simulink model "receiver"  (R2014a)
settings: Solver=ode45  StartTime=0.0  StopTime=1  RelTol=1e-3
values from neighbouring files (symbols this model uses):
  FrameTime_CP = 4e-06    [Ofdm_Parameters.mat]
  qpsktxrxOFDM =     [Ofdm_Parameters.mat]
libraries: commdigbbndam3 x2, simulink x1, commcrc2 x1, commblkintrlv2 x1, commsdrhw_v2 x1, dspsrcs4 x1
settings Model: Creator=root  LastModifiedBy=root

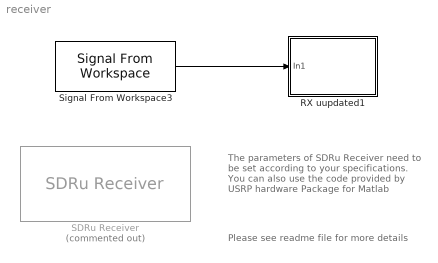
== system receiver ==
  note: Please see readme file for more details
  note: The parameters of SDRu Receiver need to be set according to your specifications. You can also use the code provided by USRP hardware Package for Matlab
  RX uupdated1 : Subsystem
      mask Display: disp('ReCeIvEr')
  SDRu Receiver : commsdrhw_v2/SDRu Receiver  Commented=on  rxtx=rx  USRP2_IP='192.168.10.2'  centerFrequency=2.45e9  centerFrequencySrc=Dialog  loOffset=0  loOffsetSrc=Dialog  gain=32  gainSrc=Dialog  decimInterp=512  decimInterpSrc=Dialog  USRP2_IP_NUM=[49 57 50 46 49 54 56 46 49 48 46 50]  frameLength=362  outputDatatype=int16  overrunUnderrunPort=off  sampleTime=1  HOST_DATA_PORT=0  HOST_CONTROL_PORT=0  USRP2_DATA_PORT=0  USRP2_CONTROL_PORT=0  bufferMode=Continuous streaming  EnableBurstMode=off  NumFramesInBurst=100
  Signal From Workspace3 : dspsrcs4/Signal From Workspace  X=corupt  Ts=2*FrameTime_CP/(qpsktxrxOFDM.OfdmSymbolSize)  nsamps=qpsktxrxOFDM.OfdmSymbolSize  OutputAfterFinalValue=Cyclic repetition  ignoreOrWarnInputAndFrameLengths=off
  wires:
  Signal From Workspace3/1 -> RX uupdated1/1(In1)

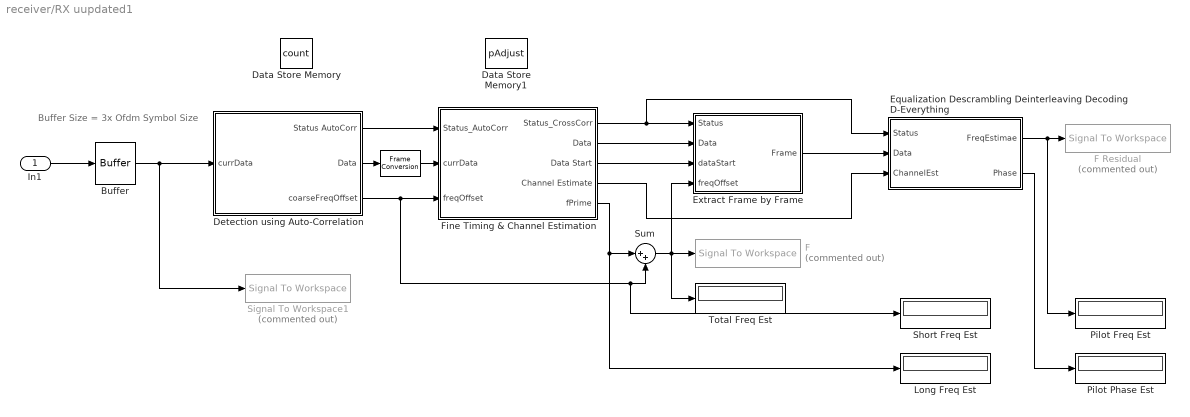
== system receiver/RX uupdated1 ==
  note: Buffer Size = 3x Ofdm Symbol Size
  In1 : Inport
  " " : FrameConversion
  Buffer : Buffer  N=qpsktxrxOFDM.OfdmSymbolSize * 3  V=qpsktxrxOFDM.OfdmSymbolSize * 2  TreatMby1Signals=One channel
  Data Store Memory : DataStoreMemory  DataStoreName=count  OutMin=0  OutMax=qpsktxrxOFDM.CounterLimit  OutDataTypeStr=double
  Data Store Memory1 : DataStoreMemory  DataStoreName=pAdjust  OutMin=0  OutMax=16  OutDataTypeStr=double
  Detection using Auto-Correlation : Subsystem
  Equalization Descrambling Deinterleaving Decoding D-Everything : Subsystem
  Extract Frame by Frame : Subsystem
  F : SignalToWorkspace  Commented=on  VariableName=freqEstTotal
      settings: CopyFcn=dspblkcopystw(gcbh);
  F Residual : SignalToWorkspace  Commented=on  VariableName=freqEstPilot
      settings: CopyFcn=dspblkcopystw(gcbh);
  Fine Timing & Channel Estimation : Subsystem
  Long Freq Est : Display
  Pilot Freq Est : Display
  Pilot Phase Est : Display
  Short Freq Est : Display
  Signal To Workspace1 : SignalToWorkspace  Commented=on  VariableName=xxx
      settings: CopyFcn=dspblkcopystw(gcbh);  Save2DSignal=3-D array (concatenate along third dimension)
  Sum : Sum  Inputs=|++
  Total Freq Est : Display
  wires:
  In1/1 -> Buffer/1
  Detection using Auto-Correlation/1(Status AutoCorr) -> Fine Timing & Channel Estimation/1(Status_AutoCorr)
  Detection using Auto-Correlation/2(Data) -> " "/1
  Buffer/1 -> Signal To Workspace1/1, Detection using Auto-Correlation/1(currData)
  " "/1 -> Fine Timing & Channel Estimation/2(currData)
  Fine Timing & Channel Estimation/2(Data) -> Extract Frame by Frame/2(Data)
  Fine Timing & Channel Estimation/3(Data Start) -> Extract Frame by Frame/3(dataStart)
  Extract Frame by Frame/1(Frame) -> Equalization Descrambling Deinterleaving Decoding D-Everything/2(Data)
  Fine Timing & Channel Estimation/4(Channel Estimate) -> Equalization Descrambling Deinterleaving Decoding D-Everything/3(ChannelEst)
  Fine Timing & Channel Estimation/1(Status_CrossCorr) -> Extract Frame by Frame/1(Status), Equalization Descrambling Deinterleaving Decoding D-Everything/1("Status ")
  Fine Timing & Channel Estimation/5(fPrime) -> Sum/1, Long Freq Est/1
  Detection using Auto-Correlation/3(coarseFreqOffset) -> Short Freq Est/1, Sum/2, Fine Timing & Channel Estimation/3(freqOffset)
  Equalization Descrambling Deinterleaving Decoding D-Everything/2(Phase) -> Pilot Phase Est/1
  Equalization Descrambling Deinterleaving Decoding D-Everything/1(FreqEstimae) -> F Residual/1, Pilot Freq Est/1
  Sum/1 -> Total Freq Est/1, F/1, Extract Frame by Frame/4(freqOffset)

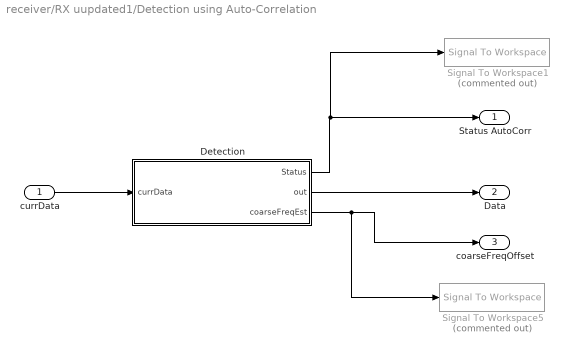
== system receiver/RX uupdated1/Detection using Auto-Correlation ==
  currData : Inport
  Detection : MATLAB Function
  Signal To Workspace1 : SignalToWorkspace  Commented=on  VariableName=StatusAutoCorr
      settings: CopyFcn=dspblkcopystw(gcbh);
  Signal To Workspace5 : SignalToWorkspace  Commented=on  VariableName=FreqEst
      settings: CopyFcn=dspblkcopystw(gcbh);
  Status AutoCorr : Outport
  Data : Outport  Port=2
  coarseFreqOffset : Outport  Port=3
  wires:
  Detection/3(coarseFreqEst) -> coarseFreqOffset/1, Signal To Workspace5/1
  Detection/1(Status) -> Signal To Workspace1/1, Status AutoCorr/1
  Detection/2(out) -> Data/1
  currData/1 -> Detection/1(currData)

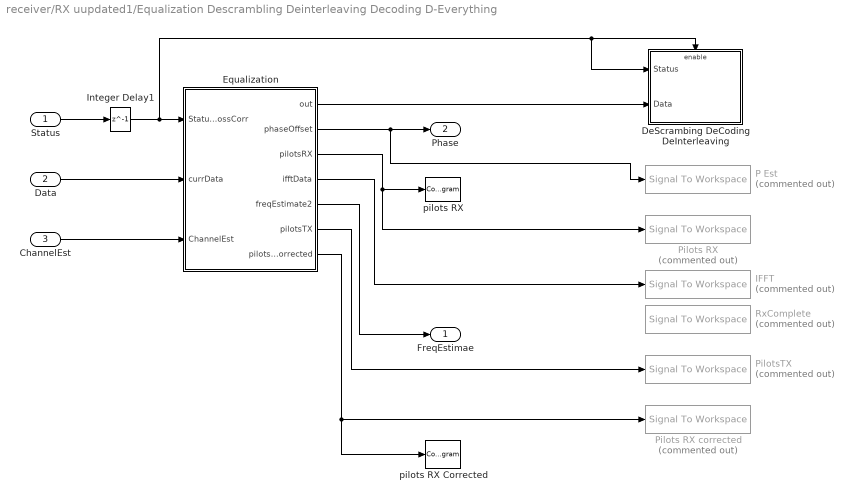
== system receiver/RX uupdated1/Equalization Descrambling Deinterleaving Decoding D-Everything ==
  "Status " : Inport
  Data : Inport  Port=2
  ChannelEst : Inport  Port=3
  DeScrambing DeCoding DeInterleaving : Subsystem
  Equalization : MATLAB Function
  IFFT : SignalToWorkspace  Commented=on  VariableName=iFFtData
      settings: CopyFcn=dspblkcopystw(gcbh);  Save2DSignal=3-D array (concatenate along third dimension)
  Integer Delay1 : Delay  DelayLength=1  InputProcessing=Inherited
  P Est : SignalToWorkspace  Commented=on  VariableName=phaseEst
      settings: CopyFcn=dspblkcopystw(gcbh);
  Pilots RX : SignalToWorkspace  Commented=on  VariableName=pilotsRX
      settings: CopyFcn=dspblkcopystw(gcbh);
  Pilots RX corrected : SignalToWorkspace  Commented=on  VariableName=pilotsRX1
      settings: CopyFcn=dspblkcopystw(gcbh);
  PilotsTX : SignalToWorkspace  Commented=on  VariableName=pilotsTX
      settings: CopyFcn=dspblkcopystw(gcbh);
  RxComplete : SignalToWorkspace  Commented=on  VariableName=RxComplete
      settings: CopyFcn=dspblkcopystw(gcbh);  Save2DSignal=3-D array (concatenate along third dimension)
  pilots RX : ConstellationDiagram  Tag=ScatterPlot
  pilots RX Corrected : ConstellationDiagram  Tag=ScatterPlot
  FreqEstimae : Outport
  Phase : Outport  Port=2
  wires:
  ChannelEst/1 -> Equalization/3(ChannelEst)
  Data/1 -> Equalization/2(currData)
  "Status "/1 -> Integer Delay1/1
  Integer Delay1/1 -> DeScrambing DeCoding DeInterleaving/1(Status), DeScrambing DeCoding DeInterleaving/Enable, Equalization/1(Status_CrossCorr)
  Equalization/2(phaseOffset) -> Phase/1, P Est/1
  Equalization/3(pilotsRX) -> Pilots RX/1, pilots RX/1
  Equalization/6(pilotsTX) -> PilotsTX/1
  Equalization/7(pilotsRX_corrected) -> Pilots RX corrected/1, pilots RX Corrected/1
  Equalization/4(ifftData) -> IFFT/1
  Equalization/1(out) -> DeScrambing DeCoding DeInterleaving/2(Data)
  ? -> RxComplete/1
  Equalization/5(freqEstimate2) -> FreqEstimae/1

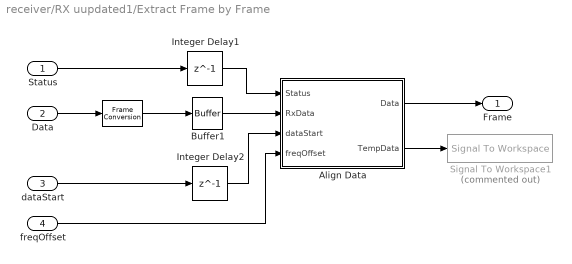
== system receiver/RX uupdated1/Extract Frame by Frame ==
  Status : Inport
  Data : Inport  Port=2
  dataStart : Inport  Port=3
  freqOffset : Inport  Port=4
  " " : FrameConversion
  Align Data : MATLAB Function  TreatAsAtomicUnit=on
  Buffer1 : Buffer  N=qpsktxrxOFDM.OfdmSymbolSize * 3  TreatMby1Signals=One channel
  Integer Delay1 : Delay  DelayLength=1  InputProcessing=Inherited
  Integer Delay2 : Delay  DelayLength=1  InputProcessing=Inherited
  Signal To Workspace1 : SignalToWorkspace  Commented=on  VariableName=TempData
      settings: CopyFcn=dspblkcopystw(gcbh);  Save2DSignal=3-D array (concatenate along third dimension)
  Frame : Outport
  wires:
  Align Data/1(Data) -> Frame/1
  Data/1 -> " "/1
  " "/1 -> Buffer1/1
  dataStart/1 -> Integer Delay2/1
  Status/1 -> Integer Delay1/1
  Integer Delay1/1 -> Align Data/1(Status)
  Buffer1/1 -> Align Data/2(RxData)
  freqOffset/1 -> Align Data/4(freqOffset)
  Align Data/2(TempData) -> Signal To Workspace1/1
  Integer Delay2/1 -> Align Data/3(dataStart)

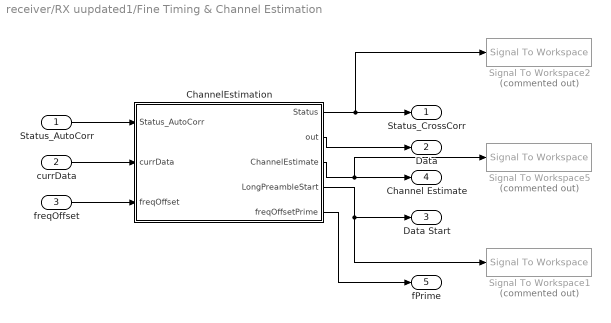
== system receiver/RX uupdated1/Fine Timing & Channel Estimation ==
  Status_AutoCorr : Inport
  currData : Inport  Port=2
  freqOffset : Inport  Port=3
  ChannelEstimation : MATLAB Function
  Signal To Workspace1 : SignalToWorkspace  Commented=on  VariableName=DataStart
      settings: CopyFcn=dspblkcopystw(gcbh);
  Signal To Workspace2 : SignalToWorkspace  Commented=on  VariableName=StatusCrossCorr
      settings: CopyFcn=dspblkcopystw(gcbh);
  Signal To Workspace5 : SignalToWorkspace  Commented=on  VariableName=ChannelESt
      settings: CopyFcn=dspblkcopystw(gcbh);
  Status_CrossCorr : Outport
  Data : Outport  Port=2
  Data Start : Outport  Port=3
  Channel Estimate : Outport  Port=4
  fPrime : Outport  Port=5
  wires:
  currData/1 -> ChannelEstimation/2(currData)
  ChannelEstimation/2(out) -> Data/1
  ChannelEstimation/1(Status) -> Status_CrossCorr/1, Signal To Workspace2/1
  Status_AutoCorr/1 -> ChannelEstimation/1(Status_AutoCorr)
  ChannelEstimation/3(ChannelEstimate) -> Signal To Workspace5/1, Channel Estimate/1
  ChannelEstimation/4(LongPreambleStart) -> Data Start/1, Signal To Workspace1/1
  freqOffset/1 -> ChannelEstimation/3(freqOffset)
  ChannelEstimation/5(freqOffsetPrime) -> fPrime/1

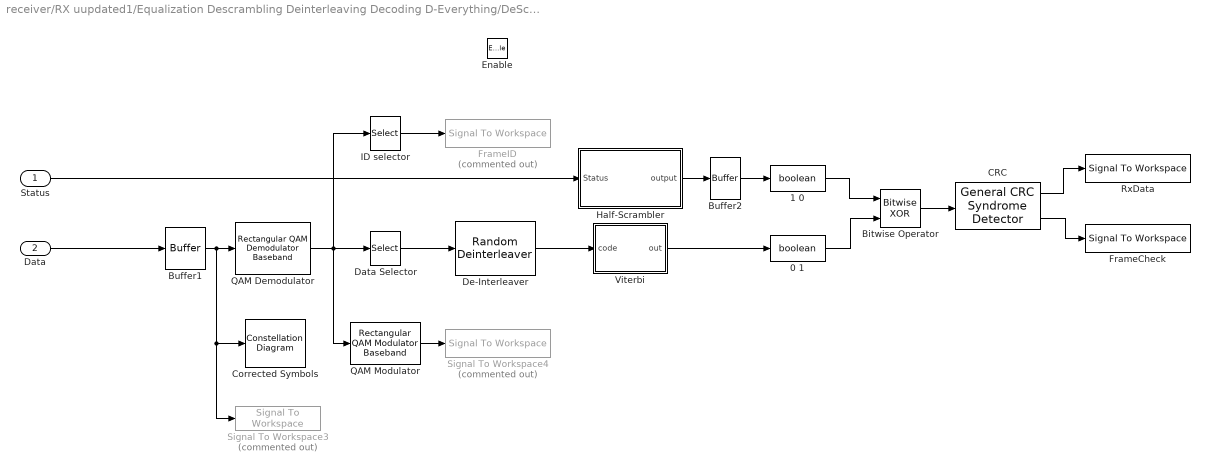
== system receiver/RX uupdated1/Equalization Descrambling Deinterleaving Decoding D-Everything/DeScrambing DeCoding DeInterleaving ==
  Status : Inport
  Data : Inport  Port=2
  Enable : EnablePort
  " QAM Modulator " : commdigbbndam3/Rectangular QAM Modulator Baseband  M=qpsktxrxOFDM.M  InType=Bit  Enc=Gray  Mapping=[0:15]  PowType=Average Power  MinDist=2  AvgPow=1  PeakPow=1  Ph=0  outDtype=double  outWordLen=16  outUDDataType=sfix(16)  outFracLenMode=Best precision  outFracLen=15
  0 1 : DataTypeConversion  OutDataTypeStr=boolean
  1 0 : DataTypeConversion  OutDataTypeStr=boolean
  Bitwise Operator : simulink/Logic and Bit Operations/Bitwise Operator  logicop=XOR  UseBitMask=off  NumInputPorts=2  BitMask=bin2dec('11011001')  BitMaskRealWorld=Stored Integer
  Buffer1 : Buffer  N=48*2  TreatMby1Signals=One channel
  Buffer2 : Buffer  N=186  TreatMby1Signals=One channel
  CRC : commcrc2/General CRC Syndrome Detector  genPoly=[1 0 0 0 0 0 0 0 1 1 1 1 1]  iniStates=0  directMethod=off  reflectInputBytes=off  reflectChecksums=off  finalXOR=0  numChecksums=1
  Corrected Symbols : ConstellationDiagram  Tag=ScatterPlot
  Data Selector : Selector  Indices=13:384
  De-Interleaver : commblkintrlv2/Random Deinterleaver  N=(qpsktxrxOFDM.DataLength + qpsktxrxOFDM.CRCLength ) * qpsktxrxOFDM.CodeRate  seed=12345
  FrameCheck : SignalToWorkspace  VariableName=FrameCheck
      settings: CopyFcn=dspblkcopystw(gcbh);
  FrameID : SignalToWorkspace  Commented=on  VariableName=FameID
      settings: CopyFcn=dspblkcopystw(gcbh);  Save2DSignal=3-D array (concatenate along third dimension)
  Half-Scrambler : MATLAB Function  TreatAsAtomicUnit=on
  ID selector : Selector  Indices=1:12
  "QAM Demodulator " : commdigbbndam3/Rectangular QAM Demodulator Baseband  M=qpsktxrxOFDM.M  PowType=Average Power  MinDist=2  AvgPow=1  PeakPow=1  Ph=0  Dec=Gray  Mapping=[0:15]  OutType=Bit  DecType=Hard decision  VarSource=Dialog  Variance=1  outDtype1=Inherit via internal rule  outDtype2=Inherit via internal rule  derotateFactorWordLen=16  denormFactorWordLen=16  prodOutWordLen=32  prodOutRoundingMode=Floor  prodOutOverflowMode=Wrap  sumWordLen=32
  RxData : SignalToWorkspace  VariableName=RxData
      settings: CopyFcn=dspblkcopystw(gcbh);  Save2DSignal=3-D array (concatenate along third dimension)
  Signal To Workspace3 : SignalToWorkspace  Commented=on  VariableName=DataSymbols
      settings: CopyFcn=dspblkcopystw(gcbh);  Save2DSignal=3-D array (concatenate along third dimension)
  Signal To Workspace4 : SignalToWorkspace  Commented=on  VariableName=DataSymbols1
      settings: CopyFcn=dspblkcopystw(gcbh);  Save2DSignal=3-D array (concatenate along third dimension)
  Viterbi : MATLAB Function  TreatAsAtomicUnit=on
  wires:
  Status/1 -> Half-Scrambler/1(Status)
  " QAM Modulator "/1 -> Signal To Workspace4/1
  "QAM Demodulator "/1 -> Data Selector/1, ID selector/1, " QAM Modulator "/1
  CRC/2 -> FrameCheck/1
  Data/1 -> Buffer1/1
  CRC/1 -> RxData/1
  Buffer1/1 -> Signal To Workspace3/1, Corrected Symbols/1, "QAM Demodulator "/1
  ID selector/1 -> FrameID/1
  Data Selector/1 -> De-Interleaver/1
  De-Interleaver/1 -> Viterbi/1(code)
  Half-Scrambler/1(output) -> Buffer2/1
  Viterbi/1(out) -> 0 1/1
  Bitwise Operator/1 -> CRC/1
  Buffer2/1 -> 1 0/1
  0 1/1 -> Bitwise Operator/2
  1 0/1 -> Bitwise Operator/1

== matlab function receiver/RX uupdated1/Fine Timing & Channel Estimation/ChannelEstimation ==
  data: Status_AutoCorr input; Status output; currData input; freqOffset input; out output; ChannelEstimate output; LongPreambleStart output; qpsktxrxOFDM parameter; count data_store_memory; freqOffsetPrime output; pAdjust data_store_memory
function [Status , out , ChannelEstimate , LongPreambleStart , freqOffsetPrime ] = channelEstimation( Status_AutoCorr , currData , freqOffset , qpsktxrxOFDM)
% THE SHORT PREAMBLES IN THE SOUBDING FRAME ARE FOLLOWED BY 10 LONG
% PREAMBLES. THE LONG PREAMBLES ARE USED FIRST TO CALCULATE REFINED START
% OF THE PACKET. CHANNEL ESTIMATE IS ALSO CALCULATED BY THE LONG PREAMBLES.
% A MORE REFINED FREQUENCY OFFSET IS ALSO CALCULATED WITH THE HELP OF LONG
% PREAMBLES.


global count pAdjust;
persistent  Status_CrossCorr ChannelEst LongPreambleStart_Est numPreambles lastPreamble endingPhase freqOffset2 freqOffsetTemp RxLongPrev;                           % No of symbols since detection

if isempty(Status_CrossCorr)
    Status_CrossCorr = 0;
    LongPreambleStart_Est = 0;
    numPreambles = 0;
    lastPreamble = 0;

    endingPhase = 0;
    freqOffset2 = 0;
    freqOffsetTemp = 0;
    RxLongPrev = complex(zeros(64,1));
end

if isempty(ChannelEst)
    ChannelEst = complex( ones(qpsktxrxOFDM.NumSubCarriers,1) );
end

if (count == qpsktxrxOFDM.CounterLimit*2)                               % time for next preambles
    count = 0;
end



% variables
longPreamble_length = 64;
Length = qpsktxrxOFDM.OfdmSymbolSize * 3; %numel(currData)


 currData2 = currData;


MaximumIndex = 0;
SecondMaximumIndex = 0;
ThirdMaximumIndex = 0;

%% PRecise Timinng via XCORR
if ( (Status_AutoCorr) && (count < 4) && (~Status_CrossCorr) ) % why equality?? 

  
    freqOffset2 = 0;
    freq = exp(1i*( 2*pi*freqOffset*(0:239).' + endingPhase ) );
    endingPhase = angle( freq(81) );
    currData = currData.*freq;
    
    ExtractedLongPreamble = qpsktxrxOFDM.Preamble(161 : 224);
    
    %% Cross Correlation    
    num_crossCorr = Length - longPreamble_length+1 ;
    CrossCorr_array = complex( zeros(1,num_crossCorr) );

    for i=1:num_crossCorr
        CrossCorr_array(i) = sum( currData(i : i + longPreamble_length - 1 ).*conj( ExtractedLongPreamble ) )...
            / sqrt( sum( ExtractedLongPreamble.*conj( ExtractedLongPreamble ) ) ...
            * sum( currData(i : i + longPreamble_length - 1 ).*conj( currData(i : i + longPreamble_length - 1 ) ) ) );
    end
    CrossCorr_array2 = abs(CrossCorr_array);
    plot(CrossCorr_array2);

    %% Checking Process
    
    [MaximumValue, MaximumIndex] = max(CrossCorr_array2);

    if (MaximumValue > .6)
    
        CrossCorr_array2 = CrossCorr_array2/MaximumValue;

        MaximumValue = 1;

        maxValue = 1;
        
        Threshold3 = 0.9;                   % detect the number of peaks
        myNumPeak=0;                        % the num of peaks in first buffer length 
        % 3 peaks and 1st maximum
        if (MaximumIndex + 64 <= 177) && (MaximumIndex + 128 <= 177) && (CrossCorr_array2(MaximumIndex + 64) >= Threshold3) && (CrossCorr_array2(MaximumIndex + 128) >= Threshold3)
            SecondMaximumIndex = MaximumIndex+64;
            SecondMaximumValue = CrossCorr_array2(SecondMaximumIndex);
            ThirdMaximumIndex = MaximumIndex+128;
            ThirdMaximumValue = CrossCorr_array2(ThirdMaximumIndex);
            myNumPeak=3;
            
            
        % 3 peaks and 2nd maximum
        elseif (MaximumIndex + 64 <= 177) && (MaximumIndex - 64 > 0) && (CrossCorr_array2(MaximumIndex + 64) >= Threshold3) && (CrossCorr_array2(MaximumIndex - 64) >= Threshold3)
            SecondMaximumIndex = MaximumIndex;
            SecondMaximumValue = CrossCorr_array2(SecondMaximumIndex);
            MaximumIndex = SecondMaximumIndex - 64;
            MaximumValue = CrossCorr_array2(MaximumIndex);
            ThirdMaximumIndex = SecondMaximumIndex + 64;
            ThirdMaximumValue = CrossCorr_array2(ThirdMaximumIndex);
            myNumPeak=3;
            
            
        % 3 peaks and 3rd maximum
        elseif (MaximumIndex - 64 > 0) && (MaximumIndex - 128 > 0) && (CrossCorr_array2(MaximumIndex - 64) >= Threshold3) && (CrossCorr_array2(MaximumIndex - 128) >= Threshold3)
            ThirdMaximumIndex = MaximumIndex;
            ThirdMaximumValue = CrossCorr_array2(ThirdMaximumIndex);
            SecondMaximumIndex = ThirdMaximumIndex - 64;
            SecondMaximumValue = CrossCorr_array2(SecondMaximumIndex);
            MaximumIndex = SecondMaximumIndex - 64;
            MaximumValue = CrossCorr_array2(MaximumIndex);
            myNumPeak=3;
            
            
        % 2 peaks and 1st maximum
        elseif (MaximumIndex + 64 <= 177) && (MaximumIndex + 128 > 177) && (CrossCorr_array2(MaximumIndex + 64) >= Threshold3)
            SecondMaximumIndex = MaximumIndex+64;
            SecondMaximumValue = CrossCorr_array2(SecondMaximumIndex);
            myNumPeak=2;
            
            
        % 2 peaks and 2nd maximum
        elseif (MaximumIndex - 64 > 0) && (CrossCorr_array2(MaximumIndex - 64) >= Threshold3)
            SecondMaximumIndex=MaximumIndex;
            SecondMaximumValue=MaximumValue;
            MaximumIndex = MaximumIndex-64;
            MaximumValue = CrossCorr_array2(MaximumIndex);
            myNumPeak=2;
            
            
        end

        threshold2 = 0.2;                      % to check that there is no value greater than threshold2 near the maximum value
        flag = 0;
        flag2 = 0;
        flag3 = 0;
        
        if (myNumPeak==2)                      % to cater multipaths
        
            freqOffsetTemp = angle( sum(currData(MaximumIndex:MaximumIndex+63) .* conj(currData(SecondMaximumIndex:SecondMaximumIndex+63))) ) / (2*pi*64 );     % 1/9 is the weight to freq offset
            
            flag=0;                                 % flag shows the number of values before MaximumIndex greater than threshold2
            for check = 1:length(CrossCorr_array2)
                
                if maxValue < threshold2
                    break
                end
                
                if ((MaximumIndex-check) >= 1) && (CrossCorr_array2(MaximumIndex-check) > threshold2)
                    flag = flag+1;
                    maxValue = CrossCorr_array2(MaximumIndex-check);
                else
                    maxValue = 0;
                end
                
            end
                flag2 = 0;
                maxValue = 1;
                for check = 1:length(CrossCorr_array2)
                    
                    if maxValue < threshold2
                        break
                    end
                    
                    if ((SecondMaximumIndex-check) >= 1) && (CrossCorr_array2(SecondMaximumIndex-check) > threshold2)
                        flag2 = flag2+1;
                        maxValue = CrossCorr_array2(SecondMaximumIndex-check);
                    else
                        maxValue = 0;
                    end
                    
                end
                
                
            
            tempFlag = max(flag , flag2);
            if (MaximumIndex-tempFlag >= 1)
                if (MaximumIndex+64 == SecondMaximumIndex) || ...
                        ( abs(CrossCorr_array2(MaximumIndex-tempFlag)-CrossCorr_array2(SecondMaximumIndex-tempFlag))/CrossCorr_array2(MaximumIndex-tempFlag) < .05 )
                    MaximumIndex = MaximumIndex - tempFlag;
                    SecondMaximumIndex = SecondMaximumIndex - tempFlag;
                else
                    fprintf('ERROR: Position mismatch')
                end
            end
            numPreambles = 2;
            LongPreambleStart_Est = MaximumIndex;
            count = 4;

        elseif (myNumPeak==3)
            
            f1 = angle( sum(currData(MaximumIndex:MaximumIndex+63) .* conj(currData(SecondMaximumIndex:SecondMaximumIndex+63))) ) / (2*pi*64 );
            f2 = angle( sum(currData(SecondMaximumIndex:SecondMaximumIndex+63) .* conj(currData(ThirdMaximumIndex:ThirdMaximumIndex+63))) ) / (2*pi*64 );
            freqOffsetTemp = (f1 + f2) / 2;
           
            
            flag=0;                                 % flag shows the number of values before MaximumIndex greater than threshold2
            for check = 1:length(CrossCorr_array2)
                
                if maxValue < threshold2
                    break
                end
                
                if ((MaximumIndex-check) >= 1) && (CrossCorr_array2(MaximumIndex-check) > threshold2)
                    flag = flag+1;
                    maxValue = CrossCorr_array2(MaximumIndex-check);
                else
                    maxValue = 0;
                end
                
            end

                flag2 = 0;
                maxValue = 1;
                for check = 1:length(CrossCorr_array2)
                    
                    if maxValue < threshold2
                        break
                    end
                    
                    if ((SecondMaximumIndex-check) >= 1) && (CrossCorr_array2(SecondMaximumIndex-check) > threshold2)
                        flag2 = flag2+1;
                        maxValue = CrossCorr_array2(SecondMaximumIndex-check);
                    else
                        maxValue = 0;
                    end
                    
                end

                flag3 = 0;
                maxValue = 1;
                for check = 1:length(CrossCorr_array2)
                    
                    if maxValue < threshold2
                        break
                    end
                    
                    if ((ThirdMaximumIndex-check) >= 1) && (CrossCorr_array2(ThirdMaximumIndex-check) > threshold2)
                        flag3 = flag3+1;
                        maxValue = CrossCorr_array2(ThirdMaximumIndex-check);
                    else
                        maxValue = 0;
                    end
                    
                end

           
            tempFlag = max(flag , flag2);
            tempFlag = max(tempFlag , flag3);
            if (MaximumIndex-tempFlag >= 1)
                if ( abs(CrossCorr_array2(MaximumIndex-tempFlag)-CrossCorr_array2(SecondMaximumIndex-tempFlag))/CrossCorr_array2(MaximumIndex-tempFlag) < .05 ) || ...
                   ( abs(CrossCorr_array2(MaximumIndex-tempFlag)-CrossCorr_array2(ThirdMaximumIndex-tempFlag))/CrossCorr_array2(MaximumIndex-tempFlag) < .05 ) || ...
                   ( abs(CrossCorr_array2(ThirdMaximumIndex-tempFlag)-CrossCorr_array2(SecondMaximumIndex-tempFlag))/CrossCorr_array2(MaximumIndex-tempFlag) < .05 ) 

                    MaximumIndex = MaximumIndex - tempFlag;
                    SecondMaximumIndex = SecondMaximumIndex - tempFlag;
                    ThirdMaximumIndex = ThirdMaximumIndex - tempFlag;
                else
                    fprintf('ERROR: Position mismatch')
                end
            end
            numPreambles = 3;
            LongPreambleStart_Est = MaximumIndex;
            count = 5;
            
        end

        %% channel estimation using long preamble
         if (count >= 4)
            
            RxLongPreamble1 = currData(LongPreambleStart_Est -pAdjust : LongPreambleStart_Est + longPreamble_length -1 -pAdjust );
            RxLongPreamble2 = currData(LongPreambleStart_Est + longPreamble_length -pAdjust : LongPreambleStart_Est + 2*longPreamble_length -1 -pAdjust );
            RxLongPrev = RxLongPreamble2;
            
            lastPreamble = LongPreambleStart_Est + 64;
            RxLongPreamble1_f = fftshift(fft(RxLongPreamble1 , qpsktxrxOFDM.NumSubCarriers));
            RxLongPreamble2_f = fftshift(fft(RxLongPreamble2 , qpsktxrxOFDM.NumSubCarriers));

            ChannelEst_1 = RxLongPreamble1_f .* conj(qpsktxrxOFDM.longPreamble_freq);    
            ChannelEst_2 = RxLongPreamble2_f .* conj(qpsktxrxOFDM.longPreamble_freq);
            ChannelEst = (ChannelEst_1 + ChannelEst_2)/10; 
            if (numPreambles == 3)
                RxLongPreamble3 = currData(LongPreambleStart_Est + 2*longPreamble_length -pAdjust : LongPreambleStart_Est + 3*longPreamble_length -1 -pAdjust );
                RxLongPreamble3_f = fftshift(fft(RxLongPreamble3 , qpsktxrxOFDM.NumSubCarriers));
                ChannelEst_3 = RxLongPreamble3_f .* conj(qpsktxrxOFDM.longPreamble_freq);
                ChannelEst = (ChannelEst_1 + ChannelEst_2 + ChannelEst_3)/10;
                lastPreamble = LongPreambleStart_Est + 128;
                RxLongPrev = RxLongPreamble3;
            end
            
            LongPreamble1_Corrected = RxLongPreamble1_f ./ (ChannelEst);
            LongPreamble2_Corrected = RxLongPreamble2_f ./ (ChannelEst);
         end
    end
    
elseif ( (Status_AutoCorr) && (numPreambles >= 2) && (count < 10) )
    
    
    freq = exp(j*( 2*pi*(freqOffset)*(0:239).' + endingPhase ) );
    endingPhase = angle( freq(81) );
    currData = currData.*freq;

    lastPreamble = lastPreamble-16;
    RxLongPreamble1 = currData(lastPreamble -pAdjust : lastPreamble + longPreamble_length -1 -pAdjust );
    
    freqTemp = angle( sum( RxLongPrev .* conj(RxLongPreamble1) ) ) / (2*pi*64 );
    RxLongPrev = RxLongPreamble1;
    freqOffsetTemp = (freqTemp/numPreambles) + freqOffsetTemp*( (numPreambles-1)/numPreambles );
    
    RxLongPreamble1_f = fftshift(fft(RxLongPreamble1 , qpsktxrxOFDM.NumSubCarriers));
    ChannelEst_1 = RxLongPreamble1_f .* conj(qpsktxrxOFDM.longPreamble_freq);
    ChannelEst = (ChannelEst_1/10 + ChannelEst);
    numPreambles = numPreambles + 1;
    if (lastPreamble <= 32) && (numPreambles < 10) 
        lastPreamble = lastPreamble+64;
        RxLongPreamble1 = currData(lastPreamble -pAdjust : lastPreamble + longPreamble_length -1 -pAdjust );

        freqTemp = angle( sum( RxLongPrev .* conj(RxLongPreamble1) ) ) / (2*pi*64 );
        RxLongPrev = RxLongPreamble1;
        freqOffsetTemp = (freqTemp/numPreambles) + freqOffsetTemp*( (numPreambles-1)/numPreambles );

        RxLongPreamble1_f = fftshift(fft(RxLongPreamble1 , qpsktxrxOFDM.NumSubCarriers));
        ChannelEst_1 = RxLongPreamble1_f .* conj(qpsktxrxOFDM.longPreamble_freq);
        ChannelEst = (ChannelEst_1/10 + ChannelEst); 
        numPreambles = numPreambles + 1;
    end
    if (numPreambles == 10)
        count = 10;                     % no of OFDM symbols (== 80 samples each) the total preamble takes
        Status_CrossCorr = 1;
        freqOffset2 = freqOffsetTemp;
    end
         
elseif ( (count >= 10) && (count <= qpsktxrxOFDM.CounterLimit*2) ) && (Status_CrossCorr) 

    
    count = count + 1;
    endingPhase = 0;
    
end

if (count == qpsktxrxOFDM.CounterLimit*2 )                           % bcoz of delay block
    Status_CrossCorr = 0;
    numPreambles = 0;
    lastPreamble = 0;
end

Status = Status_CrossCorr;
LongPreambleStart = lastPreamble;

ChannelEstimate = complex( ones(qpsktxrxOFDM.NumSubCarriers , 1) );
ChannelEstimate = ChannelEst;

freqOffsetPrime = freqOffsetTemp;

out = complex(zeros(Length,1));
out = currData2;


end

== matlab function receiver/RX uupdated1/Detection using Auto-Correlation/Detection ==
  data: Status output; currData input; out output; qpsktxrxOFDM parameter; coarseFreqEst output; count data_store_memory
function [Status , out , coarseFreqEst ] = detection( currData , qpsktxrxOFDM)

% THE SIGNAL DETECTION IS PERFORMED USING AUTOCORRELATION APPROACH OF
% PREAMBLES. 10 SHORT PREAMBLES ARE PRESENT IN THE START OF EACH SOUNDING
% FRAME. THE RECEIVER CALCULATES THE ROUGH START OF THE PACKET AND
% CALCULATES THE COARSE FREQUENCY ESTIMATE.
global count;
persistent coarseFreq Status_AutoCorr;

if isempty(coarseFreq)
   coarseFreq = 0;
end

if isempty(Status_AutoCorr)
    Status_AutoCorr = 0;
end


% variables
shortPreamble_length = 16;
Length = qpsktxrxOFDM.OfdmSymbolSize * 3; %numel(currData)

%% Packet Detection via ACORR
if (~Status_AutoCorr) 
    
    %% Auto Correlation
    AutoCorr_array2=complex(zeros(1,Length - 2*(shortPreamble_length)+1 ));

    for j=0:length(currData)-2*(shortPreamble_length)
          AutoCorr_array2(j+1) = sum( currData(j+1 : j + shortPreamble_length).*conj(currData(j+1+shortPreamble_length: j + shortPreamble_length+shortPreamble_length )) )...
              / sqrt( sum( currData(j+1 : j + shortPreamble_length).*conj(currData(j+1 : j + shortPreamble_length)) ) * ...
              sum(conj(currData(j+1+shortPreamble_length: j + shortPreamble_length+shortPreamble_length )).*currData(j+1+shortPreamble_length: j + shortPreamble_length+shortPreamble_length )) );
    end
    AutoCorr_array = abs(AutoCorr_array2);
    [maxValue , PacketStart_Esti] = max(AutoCorr_array);

    %% Checking Process
    AutoCorr_array = (AutoCorr_array) / maxValue;                       %normalize
    plot(AutoCorr_array);
    threshold = 0.8 ;%* maxValue;
    shortPreamble_Est = find(AutoCorr_array > threshold);               %gives positions in outputs
    
    num = numel(shortPreamble_Est);                                     % 7 controls the size of pleateu u r observing
    if (num >= 7*shortPreamble_length + 1 )
        Status_AutoCorr = 1;
        check = shortPreamble_Est(2:num) - shortPreamble_Est(1:num-1);  %should be all 1's in correct case
        check = check.^2;                                               % remain as one in correct case
        if sum(check) > (num - 1)
            Status_AutoCorr = 0;
        end
    end

    
    %% If Short Verified then proceed. (once every 100 or so frames (controlled by counter at TX) )
    if (Status_AutoCorr) 


        coarseFreq = angle( sum( AutoCorr_array2(shortPreamble_Est(10:end)) ) ) / (2*pi*shortPreamble_length);
        
    end

elseif (Status_AutoCorr)
    
    if (count == qpsktxrxOFDM.CounterLimit*2 - 1)
        Status_AutoCorr = 0;
    end
    
end


coarseFreqEst = coarseFreq;
Status = Status_AutoCorr;

out = complex(zeros(Length,1));
out = currData;

end

== matlab function receiver/RX uupdated1/Equalization Descrambling Deinterleaving Decoding D-Everything/Equalization ==
  data: Status_CrossCorr input; currData input; ChannelEst input; out output; qpsktxrxOFDM parameter; count data_store_memory; phaseOffset output; pilotsRX output; ifftData output; freqEstimate2 output; pilotsTX output; pilotsRX_corrected output; pAdjust data_store_memory
function [out , phaseOffset , pilotsRX , ifftData  , freqEstimate2 , pilotsTX , pilotsRX_corrected]    = Equalization( Status_CrossCorr , currData , ChannelEst , qpsktxrxOFDM)
% THIS BLOCK PERFORMS CHANNEL EQUALIZATION AND PHASE OFFSET CORRECTION BETWEEN TWO
% SOUNDING FRAMES. THE PHASE OFFSET CORRECTION IS PERFORMEND USING THE
% PHASE OFFSETS EXTRACTED FROM PILOTS. EQUALIZATION IS PERFORMED USING THE CHANNEL
% ESTIMATES CALCULATED FROM LONG PREAMBLES IN "FINE TIMING AND CHANNEL
% ESTIMATE BLOCK"


global pAdjust;
persistent state pilotsPrev freqEstimate endPhase freqFIFO ;

if isempty(state)
   state = [1 1 1 1 1 1 0];     % actual initial =  [1 1 1 1 1 1 1] but for skipping signal packet i evaluate first iteration by hand
   pilotsPrev = complex( zeros(4,1) );
   freqEstimate = 0;
   endPhase = 0;
   freqFIFO = zeros(1,10);
end

out = complex( zeros(qpsktxrxOFDM.NumDataSubCarriers , 1) );
pilotsRX = complex(zeros(4,1));
pilotsRX_corrected = complex(zeros(4,1));
pilotsTX = complex(zeros(4,1));
phaseOffset=0;
freqEstimate2 = 0;      % for output only

%% freq correction from pilots

ifftData = complex(zeros(64,1));    
RxComplete = complex(zeros(64,1));
RxComplete2 = complex(zeros(64,1));

if (Status_CrossCorr)
    
    %% Actual Pilot generation
    bitLength = 1;

    pilot = zeros(bitLength,1);
    poly = state;

    for i = 1:bitLength
        pilot(i) = mod(poly(1) + poly(4) , 2);
        poly = [poly(2:end) pilot(i)];
    end

    if pilot == 0
        pilot = 1;
    elseif pilot == 1
        pilot = -1;
    end    

    state = poly;

    pilotsTX = [1 1 1 -1].';
    pilotsTX = pilotsTX .* pilot;
    
    %% FFt
    RxComplete = currData( qpsktxrxOFDM.NumSubCarriers - qpsktxrxOFDM.NumDataSubCarriers +1 -pAdjust : end -pAdjust );%fftData;    
    RxComplete2 = RxComplete;
    ifftData = fftshift( fft(RxComplete , qpsktxrxOFDM.NumSubCarriers) ); 

    ifftData = ifftData ./ ChannelEst;

    %% Pilot and data separation
    completeDatatemp = complex(zeros(48,1));

    pilotsRX(1) = ifftData(12);
    pilotsRX(2) = ifftData(26);
    pilotsRX(3) = ifftData(40);
    pilotsRX(4) = ifftData(54);
    
    % frequency caluculation from pilots
    freqEstimateTemp = conj( pilotsRX.*pilotsTX ) .* pilotsPrev ;
    freqEstimate2 = angle( sum(freqEstimateTemp) ) / (2*pi*80);
    freqFIFO = [freqEstimate2 freqFIFO(1:end-1)];
    freqEstimate = mean(freqFIFO);
    
    % phase caluculation from pilots
    phaseOffset = angle( sum( (pilotsRX.*conj(pilotsTX)) ) );
    
    completeDatatemp(1:5) = ifftData(7:11);
    
    completeDatatemp(6:18) = ifftData(13:25);
    
    completeDatatemp(19:24) = ifftData(27:32);
    
    completeDatatemp(25:30) = ifftData(34:39);

    completeDatatemp(31:43) = ifftData(41:53);
    
    completeDatatemp(44:48) = ifftData(55:59);

    completeDatatemp=completeDatatemp*exp(-1i*phaseOffset);      % pilot corrction
    
    out = completeDatatemp;
    
    pilotsRX_corrected = pilotsRX.*exp(-1i*phaseOffset);

    pilotsPrev = pilotsRX.*pilotsTX;

else
    
    pilotsPrev = zeros(4,1);
    
end
    
    
end

== matlab function receiver/RX uupdated1/Equalization Descrambling Deinterleaving Decoding D-Everything/DeScrambing DeCoding DeInterleaving/Half-Scrambler ==
  data: Status input; output output
function output  = scrambler(Status )

persistent state;

if isempty(state)
   state = [1 0 1 1 1 0 1];
end

bitLength = (174 + 12)/2;   %length + CRC

output = zeros(bitLength,1);

if (Status)
    poly = state;

    for i = 1:bitLength
        output(i) = mod(poly(1) + poly(4) , 2);
        poly = [poly(2:end) output(i)];
    end


    state = poly;
end

end

== matlab function receiver/RX uupdated1/Equalization Descrambling Deinterleaving Decoding D-Everything/DeScrambing DeCoding DeInterleaving/Viterbi ==
  data: code input; out output
function out  = deconv( code)

coder.extrinsic('vitdec');
trellis = struct('numInputSymbols',2,'numOutputSymbols',4,... % define trellis faster
'numStates',8,'nextStates',[0 4;0 4;1 5;1 5;2 6;2 6;3 7;3 7],...
'outputs',[0 3;3 0;3 0;0 3;1 2;2 1;2 1;1 2]);

tblen = 25;

out = zeros(186,1);
out = vitdec(code,trellis,tblen,'trunc','hard');

end

== matlab function receiver/RX uupdated1/Extract Frame by Frame/Align Data ==
  data: Status input; RxData input; dataStart input; Data output; freqOffset input; TempData output
function [Data , TempData]= aligndata( Status , RxData , dataStart , freqOffset)
% Extract data from the buffered RxData, using the delay to find the frame 

persistent endphase freqL;

if isempty(endphase)    
    endphase = 0;
    freqL = 0;
end

Data = complex(zeros(80,1));
TempData = complex(zeros(80,1));

if Status
    freqL = freqOffset;             %% updated only when both est from short and long have been gotten
    out = RxData( dataStart + 64 - 80 : dataStart + 64 - 80 + 79 );
    Data = out(1:80);
    TempData = Data;
end

freq = exp(1i*(2*pi*freqL*(1:80).' + endphase));
 Data = Data.*freq;
endphase = angle( freq(end) );
